simulink model "Rebuild"  (R2024b)
settings: Solver=VariableStepAuto  StartTime=0.0  StopTime=12  RelTol=1e-3
values from neighbouring files (symbols this model uses):
  A = 1.1    [RT14e_Parameters.m]    (also in RT15e_Parameters.m = 1.088; RT15evo_Parameters.m = 1.088)
  Aero_balance = 55    [RT14e_Parameters.m]    (also in RT15e_Parameters.m; RT15evo_Parameters.m)
  Aeromaps_ON = 0    [SIM_setup.m]
  air_density = 1.2    [SIM_setup.m]
  Balance_FW = Data_FW_STD(1:end,2)    [RT15e_Parameters.m]    (also in RT15evo_Parameters.m)
  Balance_R_11 = Data_R_11(1:end,2)    [RT15e_Parameters.m]    (also in RT15evo_Parameters.m)
  Br_coef_of_friction_F = 0.33    [RT14e_Parameters.m]    (also in RT15e_Parameters.m; RT15evo_Parameters.m)
  Br_coef_of_friction_R = 0.33    [RT14e_Parameters.m]    (also in RT15e_Parameters.m; RT15evo_Parameters.m)
  Br_pistons_area_F = 3617.26/1e6    (= 0.00361726)    [RT14e_Parameters.m]    (also in RT15e_Parameters.m; RT15evo_Parameters.m)
  Br_pistons_area_R = 2026.83/1e6    (= 0.00202683)    [RT14e_Parameters.m]    (also in RT15e_Parameters.m; RT15evo_Parameters.m)
  CdA = 1.31*A    (= 1.441)    [RT14e_Parameters.m]    (also in RT15e_Parameters.m = 1.700544; RT15evo_Parameters.m = 1.700544)
  CdA_FW = Data_FW_STD(1:end,3)    [RT15e_Parameters.m]    (also in RT15evo_Parameters.m)
  CdA_R_11 = Data_R_11(1:end,3)    [RT15e_Parameters.m]    (also in RT15evo_Parameters.m)
  ClA = 3.3*A    (= 3.63)    [RT14e_Parameters.m]    (also in RT15e_Parameters.m = 4.36288; RT15evo_Parameters.m = 4.36288)
  ClA_FW = Data_FW_STD(1:end,4)    [RT15e_Parameters.m]    (also in RT15evo_Parameters.m)
  ClA_R_11 = Data_R_11(1:end,4)    [RT15e_Parameters.m]    (also in RT15evo_Parameters.m)
  CoG_z = 0.35    [RT14e_Parameters.m]    (also in RT15e_Parameters.m = 0.28495; RT15evo_Parameters.m = 0.28495)
  Default_Fz_FL = Default_Fz_F/2 + (Default_Fz_F*CoG_y/Track_Front)    [RT14e_Parameters.m]    (also in RT15e_Parameters.m; RT15evo_Parameters.m)
  Default_Fz_FR = Default_Fz_F/2 - (Default_Fz_F*CoG_y/Track_Front)    [RT14e_Parameters.m]    (also in RT15e_Parameters.m; RT15evo_Parameters.m)
  Default_Fz_RL = Default_Fz_R/2 + (Default_Fz_R*CoG_y/Track_Rear)    [RT14e_Parameters.m]    (also in RT15e_Parameters.m; RT15evo_Parameters.m)
  Default_Fz_RR = Default_Fz_R/2 - (Default_Fz_R*CoG_y/Track_Rear)    [RT14e_Parameters.m]    (also in RT15e_Parameters.m; RT15evo_Parameters.m)
  Effective_br_disk_r_F = 0.0905    [RT14e_Parameters.m]    (also in RT15e_Parameters.m; RT15evo_Parameters.m)
  Effective_br_disk_r_R = 0.0895    [RT14e_Parameters.m]    (also in RT15e_Parameters.m; RT15evo_Parameters.m)
  Front_brake_balance = 0.0    (= 0)    [RT14e_Parameters.m]    (also in RT15e_Parameters.m; RT15evo_Parameters.m)
  Front_brake_pump_area = 153.94    [RT14e_Parameters.m]    (also in RT15e_Parameters.m; RT15evo_Parameters.m)
  Front_desired_brake_p_balance = 0.6    [RT14e_Parameters.m]    (also in RT15e_Parameters.m; RT15evo_Parameters.m)
  FW_Setup = Data_FW_STD(1:end,1)    [RT15e_Parameters.m]    (also in RT15evo_Parameters.m)
  Fx = Data_Fx(2:end,3:end)    [RT14e_Parameters.m]    (also in RT15e_Parameters.m; RT15evo_Parameters.m)
  Fy = Data_Fy(2:end,3:end)    [RT14e_Parameters.m]    (also in RT15e_Parameters.m; RT15evo_Parameters.m)
  Fz = Data_Fy(2:end,2)    [RT14e_Parameters.m]    (also in RT15e_Parameters.m; RT15evo_Parameters.m)
  g = 9.81    [SIM_setup.m]
  Gear_ratio = 12.9    [RT14e_Parameters.m]    (also in RT15e_Parameters.m; RT15evo_Parameters.m)
  Iz_wehicle = 120    [RT14e_Parameters.m]    (also in RT15e_Parameters.m; RT15evo_Parameters.m)
  Iz_wheel = 0.15    [RT14e_Parameters.m]    (also in RT15e_Parameters.m; RT15evo_Parameters.m)
  Lf = Wheelbase - CoG_x    (= 0.77)    [RT14e_Parameters.m]    (also in RT15e_Parameters.m = 0.7504; RT15evo_Parameters.m = 0.7504)
  LLTD = 0.45    [RT14e_Parameters.m]    (also in RT15e_Parameters.m = 0.55; RT15evo_Parameters.m = 0.55)
  Lock_brake_balance = false    [RT14e_Parameters.m]    (also in RT15e_Parameters.m; RT15evo_Parameters.m)
  Lr = Wheelbase - Lf    (= 0.755)    [RT14e_Parameters.m]    (also in RT15e_Parameters.m = 0.7746; RT15evo_Parameters.m = 0.7746)
  Mass = Vehicle_mass + Driver_mass    (= 290)    [RT14e_Parameters.m]    (also in RT15e_Parameters.m = 265; RT15evo_Parameters.m)
  Motor_maximum_power = 35366    [RT14e_Parameters.m]    (also in RT15e_Parameters.m; RT15evo_Parameters.m)
  RB_torque_setting_1 = -2    [RT14e_Parameters.m]    (also in RT15e_Parameters.m; RT15evo_Parameters.m)
  RB_torque_setting_10 = -20    [RT14e_Parameters.m]    (also in RT15e_Parameters.m; RT15evo_Parameters.m)
  RB_torque_setting_2 = -4    [RT14e_Parameters.m]    (also in RT15e_Parameters.m; RT15evo_Parameters.m)
  RB_torque_setting_3 = -6    [RT14e_Parameters.m]    (also in RT15e_Parameters.m; RT15evo_Parameters.m)
  RB_torque_setting_4 = -8    [RT14e_Parameters.m]    (also in RT15e_Parameters.m; RT15evo_Parameters.m)
  RB_torque_setting_5 = -10    [RT14e_Parameters.m]    (also in RT15e_Parameters.m; RT15evo_Parameters.m)
  RB_torque_setting_6 = -12    [RT14e_Parameters.m]    (also in RT15e_Parameters.m; RT15evo_Parameters.m)
  RB_torque_setting_7 = -14    [RT14e_Parameters.m]    (also in RT15e_Parameters.m; RT15evo_Parameters.m)
  RB_torque_setting_8 = -16    [RT14e_Parameters.m]    (also in RT15e_Parameters.m; RT15evo_Parameters.m)
  RB_torque_setting_9 = -18    [RT14e_Parameters.m]    (also in RT15e_Parameters.m; RT15evo_Parameters.m)
  Rear_brake_pump_area = 198.56    [RT14e_Parameters.m]    (also in RT15e_Parameters.m; RT15evo_Parameters.m)
  Roll_Angle_11 = Data_R_11(1:end,1)    [RT15e_Parameters.m]    (also in RT15evo_Parameters.m)
  SA = Data_Fy(1,3:end)    [RT14e_Parameters.m]    (also in RT15e_Parameters.m; RT15evo_Parameters.m)
  SR = Data_Fx(1,3:end)    [RT14e_Parameters.m]    (also in RT15e_Parameters.m; RT15evo_Parameters.m)
  start_acc_x = double(start_acc_x_ts.Data)    [SIM_setup.m]
  start_acc_y = double(start_acc_y_ts.Data)    [SIM_setup.m]
  start_time = 1188    [SIM_setup.m]
  start_velocity_x = double(start_velocity_x_ts.Data)    [SIM_setup.m]
  start_velocity_y = double(start_velocity_y_ts.Data)    [SIM_setup.m]
  start_yaw_acc = double(start_yaw_acc_ts.Data)    [SIM_setup.m]
  start_yaw_rate = double(start_yaw_rate_ts.Data)    [SIM_setup.m]
  Static_Camber_FL = 0    [RT14e_Parameters.m]    (also in RT15e_Parameters.m; RT15evo_Parameters.m)
  Static_Camber_FR = 0    [RT14e_Parameters.m]    (also in RT15e_Parameters.m; RT15evo_Parameters.m)
  Static_Camber_RL = 0    [RT14e_Parameters.m]    (also in RT15e_Parameters.m; RT15evo_Parameters.m)
  Static_Camber_RR = 0    [RT14e_Parameters.m]    (also in RT15e_Parameters.m; RT15evo_Parameters.m)
  Static_Toe_FL = 0    [RT14e_Parameters.m]    (also in RT15e_Parameters.m; RT15evo_Parameters.m)
  Static_Toe_FR = 0    [RT14e_Parameters.m]    (also in RT15e_Parameters.m; RT15evo_Parameters.m)
  Static_Toe_RL = 0    [RT14e_Parameters.m]    (also in RT15e_Parameters.m; RT15evo_Parameters.m)
  Static_Toe_RR = 0    [RT14e_Parameters.m]    (also in RT15e_Parameters.m; RT15evo_Parameters.m)
  Steering_Angle_FL = Data_Steering(1:end,2)    [RT14e_Parameters.m]    (also in RT15e_Parameters.m; RT15evo_Parameters.m)
  Steering_Angle_FR = Data_Steering(1:end,3)    [RT14e_Parameters.m]    (also in RT15e_Parameters.m; RT15evo_Parameters.m)
  Steering_Wheel_Angle = Data_Steering(1:end,1)    [RT14e_Parameters.m]    (also in RT15e_Parameters.m; RT15evo_Parameters.m)
  Tire_radius = 0.203    [RT14e_Parameters.m]    (also in RT15e_Parameters.m; RT15evo_Parameters.m)
  Torque_limit_2 = Motor_maximum_torque*0.2    (= 5.82)    [RT14e_Parameters.m]    (also in RT15e_Parameters.m; RT15evo_Parameters.m)
  Torque_limit_3 = Motor_maximum_torque*0.3    (= 8.73)    [RT14e_Parameters.m]    (also in RT15e_Parameters.m; RT15evo_Parameters.m)
  Torque_limit_4 = Motor_maximum_torque*0.4    (= 11.64)    [RT14e_Parameters.m]    (also in RT15e_Parameters.m; RT15evo_Parameters.m)
  Torque_limit_5 = Motor_maximum_torque*0.5    (= 14.55)    [RT14e_Parameters.m]    (also in RT15e_Parameters.m; RT15evo_Parameters.m)
  Torque_limit_6 = Motor_maximum_torque*0.6    (= 17.46)    [RT14e_Parameters.m]    (also in RT15e_Parameters.m; RT15evo_Parameters.m)
  Torque_limit_7 = Motor_maximum_torque*0.7    (= 20.37)    [RT14e_Parameters.m]    (also in RT15e_Parameters.m; RT15evo_Parameters.m)
  Torque_limit_8 = Motor_maximum_torque*0.8    (= 23.28)    [RT14e_Parameters.m]    (also in RT15e_Parameters.m; RT15evo_Parameters.m)
  Torque_limit_9 = 29.1    [RT14e_Parameters.m]    (also in RT15e_Parameters.m; RT15evo_Parameters.m)
  Torque_limit_max = Motor_maximum_torque    (= 29.1)    [RT14e_Parameters.m]    (also in RT15e_Parameters.m; RT15evo_Parameters.m)
  Torque_limit_min = Motor_maximum_torque*0.1    (= 2.91)    [RT14e_Parameters.m]    (also in RT15e_Parameters.m; RT15evo_Parameters.m)
  Torque_limit_set = 10    [RT14e_Parameters.m]    (also in RT15e_Parameters.m; RT15evo_Parameters.m)
  Track_Front = 1.2    [RT14e_Parameters.m]    (also in RT15e_Parameters.m; RT15evo_Parameters.m)
  Track_Rear = 1.18    [RT14e_Parameters.m]    (also in RT15e_Parameters.m; RT15evo_Parameters.m)
  TV_ON = 0    [SIM_setup.m]
  TV_RB_understeer_gradient_1 = -0.5    [RT14e_Parameters.m]    (also in RT15e_Parameters.m; RT15evo_Parameters.m)
  TV_RB_understeer_gradient_10 = 0.005    [RT14e_Parameters.m]    (also in RT15e_Parameters.m; RT15evo_Parameters.m)
  TV_RB_understeer_gradient_2 = -0.1    [RT14e_Parameters.m]    (also in RT15e_Parameters.m; RT15evo_Parameters.m)
  TV_RB_understeer_gradient_3 = 0.08    [RT14e_Parameters.m]    (also in RT15e_Parameters.m; RT15evo_Parameters.m)
  TV_RB_understeer_gradient_4 = 0.06    [RT14e_Parameters.m]    (also in RT15e_Parameters.m; RT15evo_Parameters.m)
  TV_RB_understeer_gradient_5 = 0.05    [RT14e_Parameters.m]    (also in RT15e_Parameters.m; RT15evo_Parameters.m)
  TV_RB_understeer_gradient_6 = 0.04    [RT14e_Parameters.m]    (also in RT15e_Parameters.m; RT15evo_Parameters.m)
  TV_RB_understeer_gradient_7 = 0.03    [RT14e_Parameters.m]    (also in RT15e_Parameters.m; RT15evo_Parameters.m)
  TV_RB_understeer_gradient_8 = 0.02    [RT14e_Parameters.m]    (also in RT15e_Parameters.m; RT15evo_Parameters.m)
  TV_RB_understeer_gradient_9 = 0.01    [RT14e_Parameters.m]    (also in RT15e_Parameters.m; RT15evo_Parameters.m)
  TV_understeer_gradient_1 = -0.5    [RT14e_Parameters.m]    (also in RT15e_Parameters.m; RT15evo_Parameters.m)
  TV_understeer_gradient_10 = 0.002    [RT14e_Parameters.m]    (also in RT15e_Parameters.m; RT15evo_Parameters.m)
  TV_understeer_gradient_2 = -0.1    [RT14e_Parameters.m]    (also in RT15e_Parameters.m; RT15evo_Parameters.m)
  TV_understeer_gradient_3 = 0.06    [RT14e_Parameters.m]    (also in RT15e_Parameters.m; RT15evo_Parameters.m)
  TV_understeer_gradient_4 = 0.05    [RT14e_Parameters.m]    (also in RT15e_Parameters.m; RT15evo_Parameters.m)
  TV_understeer_gradient_5 = 0.04    [RT14e_Parameters.m]    (also in RT15e_Parameters.m; RT15evo_Parameters.m)
  TV_understeer_gradient_6 = 0.03    [RT14e_Parameters.m]    (also in RT15e_Parameters.m; RT15evo_Parameters.m)
  TV_understeer_gradient_7 = 0.02    [RT14e_Parameters.m]    (also in RT15e_Parameters.m; RT15evo_Parameters.m)
  TV_understeer_gradient_8 = 0.01    [RT14e_Parameters.m]    (also in RT15e_Parameters.m; RT15evo_Parameters.m)
  TV_understeer_gradient_9 = 0.005    [RT14e_Parameters.m]    (also in RT15e_Parameters.m; RT15evo_Parameters.m)
  Vx_APPS_ON = 1    [SIM_setup.m]
  Wheel_rolling_resistance = 0.055    [RT14e_Parameters.m]    (also in RT15e_Parameters.m; RT15evo_Parameters.m)
  Wheelbase = 1.525    [RT14e_Parameters.m]    (also in RT15e_Parameters.m; RT15evo_Parameters.m)
undefined symbols (not defined in the file or in its folder): Actual_Torque_Value_RL, Actual_Torque_Value_RR, aero_balance, APPS, Brake_Pressure_Front, Brake_Pressure_Rear, Cl, lateral_load_transfer_distribution, maths_GPS_Velocity, Max_Torque, rad, s, Steering_position, tire_radius, wheel_base, Wheel_Speed_RL, Wheel_Speed_RR, Xsens_MTI_670_accX, Xsens_MTI_670_accY, Xsens_MTI_670_gyrZ
libraries: simulink x30, simulink_extras x11, slpidlib x9, dspstat3 x4, slrealtimeloglib x1, aerolibconvert2 x1
(part 1 of 6)
settings Model: Creator=ciech  LastModifiedBy=ciech
settings SolverCC: ZeroCrossControl=EnableAll
settings DebuggingCC: IgnoredZcDiagnostic=none

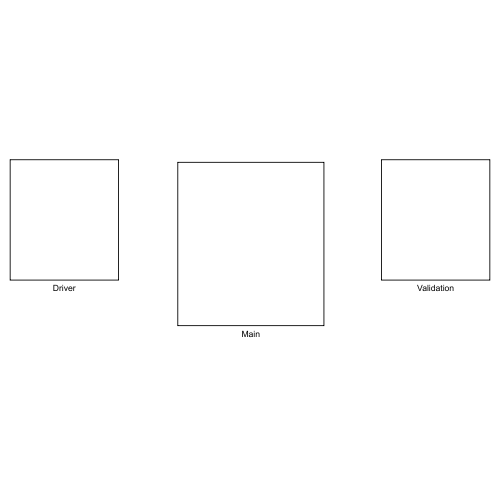
[thumbnail: Simulink's stored preview of the top-level diagram]
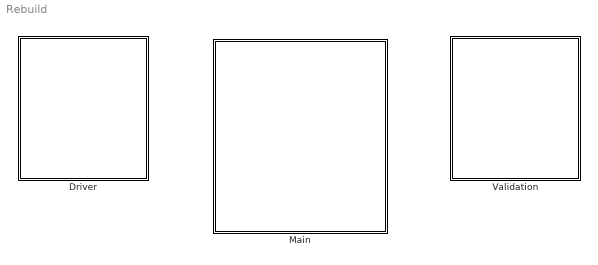
== system Rebuild ==
  Driver : Subsystem
  Main : Subsystem
  Validation : Subsystem

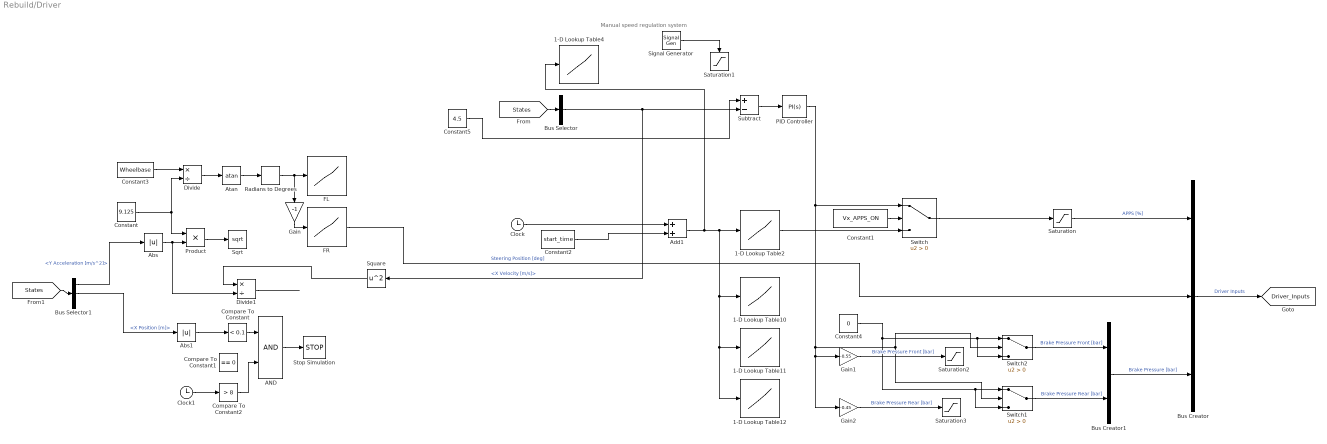
== system Rebuild/Driver ==
  note: Manual speed regulation system
  1-D Lookup Table10 : Lookup_n-D  NumberOfTableDimensions=1  BreakpointsForDimension1=Steering_position.Time  Table=Steering_position.Value  InternalRulePriority=Speed  RndMeth=Simplest
  1-D Lookup Table11 : Lookup_n-D  NumberOfTableDimensions=1  BreakpointsForDimension1=Brake_Pressure_Front.Time  Table=Brake_Pressure_Front.Value  InternalRulePriority=Speed  RndMeth=Simplest
  1-D Lookup Table12 : Lookup_n-D  NumberOfTableDimensions=1  BreakpointsForDimension1=Brake_Pressure_Rear.Time  Table=Brake_Pressure_Rear.Value  InternalRulePriority=Speed  RndMeth=Simplest
  1-D Lookup Table2 : Lookup_n-D  NumberOfTableDimensions=1  BreakpointsForDimension1=APPS.Time  Table=APPS.Value  InternalRulePriority=Speed  RndMeth=Simplest
  1-D Lookup Table4 : Lookup_n-D  NumberOfTableDimensions=1  BreakpointsForDimension1=maths_GPS_Velocity.Time  Table=maths_GPS_Velocity.Value  InternalRulePriority=Speed  RndMeth=Simplest
  AND : Logic  IconShape=distinctive  AllPortsSameDT=off  OutDataTypeStr=boolean
  Abs : Abs  SaturateOnIntegerOverflow=off
  Abs1 : Abs  SaturateOnIntegerOverflow=off
  Add1 : Sum
  Atan : Trigonometry  Operator=atan
  Bus Creator : BusCreator  Inputs=3
  Bus Creator1 : BusCreator  Inputs=2
  Bus Selector : BusSelector  OutputSignals=Velocitiy [m/s].X Velocity [m/s]
  Bus Selector1 : BusSelector  OutputSignals=Acceleration [m/s].Y Acceleration [m/s^2],Position [m].X Position [m],Position [m].Y Position [m]
  Clock : Clock
  Clock1 : Clock
  Compare To Constant : simulink/Logic and Bit Operations/Compare To Constant  relop=<  const=0.1  OutDataTypeStr=boolean
  Compare To Constant1 : simulink/Logic and Bit Operations/Compare To Constant  relop===  const=0  OutDataTypeStr=boolean
  Compare To Constant2 : simulink/Logic and Bit Operations/Compare To Constant  relop=>  const=8  OutDataTypeStr=boolean
  Constant : Constant  Value=9.125
  Constant1 : Constant  Value=Vx_APPS_ON
  Constant2 : Constant  Value=start_time
  Constant3 : Constant  Value=Wheelbase
  Constant4 : Constant  Value=0
  Constant5 : Constant  Value=4.5
  Divide : Product  Inputs=*/
  Divide1 : Product  Inputs=*/
  FL : Lookup_n-D  NumberOfTableDimensions=1  BreakpointsForDimension1=Steering_Angle_FL  Table=Steering_Wheel_Angle  InternalRulePriority=Speed  RndMeth=Simplest
  FR : Lookup_n-D  NumberOfTableDimensions=1  BreakpointsForDimension1=Steering_Angle_FR*-1  Table=Steering_Wheel_Angle  InternalRulePriority=Speed  RndMeth=Simplest
  Gain : Gain  Gain=-1
  Gain1 : Gain  Gain=-0.55
  Gain2 : Gain  Gain=-0.45
  PID Controller : slpidlib/PID Controller  Controller=PI  Form=Parallel  TimeDomain=Continuous-time  UseExternalTs=off  SampleTime=-1  IntegratorMethod=Forward Euler  FilterMethod=Forward Euler  ControllerParametersSource=internal  P=70  I=40  UseKiTs=off  D=20  UseExternalDerivativeSource=off  N=100  UseFilter=on  TunerSelectOption=Transfer Function Based (PID Tuner App)  InitialConditionSource=internal  InitialConditionForIntegrator=0  InitialConditionForFilter=0  DifferentiatorICPrevScaledInput=0  ExternalReset=none  TrackingMode=off  Kt=1  LimitOutput=off  SatLimitsSource=internal  UpperSaturationLimit=100  LowerSaturationLimit=0  LinearizeAsGain=on  AntiWindupMode=back-calculation  Kb=1  LimitIntegrator=off  UpperIntegratorSaturationLimit=inf  LowerIntegratorSaturationLimit=-inf  POutMin=[]  POutMax=[]  IOutMin=[]  IOutMax=[]  DOutMin=[]  DOutMax=[]  NOutMin=[]  NOutMax=[]  SumOutMin=[]  SumOutMax=[]  SaturationOutMin=[]  SaturationOutMax=[]  PParamMin=[]  PParamMax=[]  IParamMin=[]  IParamMax=[]  DParamMin=[]  DParamMax=[]  NParamMin=[]  NParamMax=[]  KbParamMin=[]  KbParamMax=[]  KtParamMin=[]  KtParamMax=[]  KbOutMin=[]  KbOutMax=[]  KtOutMin=[]  KtOutMax=[]  IntegratorOutMin=[]  IntegratorOutMax=[]  FilterOutMin=[]  FilterOutMax=[]  SumI1OutMin=[]  SumI1OutMax=[]  SumI2OutMin=[]  SumI2OutMax=[]  SumI3OutMin=[]  SumI3OutMax=[]  SumI4OutMin=[]  SumI4OutMax=[]  SumDOutMin=[]  SumDOutMax=[]  DifferentiatorOutMin=[]  DifferentiatorOutMax=[]  FilterDiffOutCoefMin=[]  FilterDiffOutCoefMax=[]  ReciprocalOutMin=[]  ReciprocalOutMax=[]  SumDenOutMin=[]  SumDenOutMax=[]  SumNumOutMin=[]  SumNumOutMax=[]  DivideOutMin=[]  DivideOutMax=[]  UdiffTsProdOutMin=[]  UdiffTsProdOutMax=[]  NTsProdOutMin=[]  NTsProdOutMax=[]  UintegralTsProdOutMin=[]  UintegralTsProdOutMax=[]  UngainTsProdOutMin=[]  UngainTsProdOutMax=[]  ClampingZeroOutDataTypeStr=Inherit: Inherit via back propagation  ClampingZeroOutMin=[]  ClampingZeroOutMax=[]  FilterDenConstantOutDataTypeStr=Inherit: Inherit via back propagation  FilterDenConstantOutMin=[]  FilterDenConstantOutMax=[]  PCopyOutDataTypeStr=Inherit: Inherit via back propagation  PCopyOutMin=[]  PCopyOutMax=[]  NCopyOutDataTypeStr=Inherit: Inherit via back propagation  NCopyOutMin=[]  NCopyOutMax=[]  IntegratorContinuousStateAttributes=''  IntegratorStateMustResolveToSignalObject=off  IntegratorRTWStateStorageClass=Auto  FilterContinuousStateAttributes=''  FilterStateMustResolveToSignalObject=off  FilterRTWStateStorageClass=Auto  ParallelPVariant=InternalParameters  IdealPVariant=Disabled  IVariant=InternalParameters  DVariant=Disabled  IntegratorVariant=Continuous  SatVariant=Disabled  AWVariant=Passthrough  PCopyVariant=Disabled  TRVariant=Disabled  FdbkBlocksVariant=Forward  IdealPFdbkVariant=Disabled  SatFdbkVariant=Disabled  DerivativeFilterVariant=Disabled  NVariant=Disabled  NCopyVariant=Disabled_SignalSpec  FilterICVariant=Disabled  IntegratorICVariant=InternalICs  ExternalResetVariant=Disabled  TRSumVariant=Passthrough  SumFdbkVariant=Disabled  SumVariant=Sum_PI  TsampFilterVariant=InternalTs  TsampNgainVariant=Passthrough  TsampIntegralVariant=Disabled_SignalSpec  ExternalSaturationOutDataTypeStr=Inherit: Same as second input  DerivativeSourceVariant=Disabled  PreIntVariant=InternalPreInt
  Product : Product
  Radians to Degrees : simulink_extras/Transformations/Radians to Degrees
  Saturation : Saturate  UpperLimit=100  LowerLimit=0
  Saturation1 : Saturate  UpperLimit=inf  LowerLimit=10
  Saturation2 : Saturate  UpperLimit=70  LowerLimit=0
  Saturation3 : Saturate  UpperLimit=70  LowerLimit=0
  Signal Generator : SignalGenerator  Amplitude=20  Frequency=2  Units=rad/sec
  Sqrt : Sqrt
  Square : Math  Operator=square
  Stop Simulation : Stop
  Subtract : Sum  Inputs=+-
  Switch : Switch  Criteria=u2 > Threshold  SaturateOnIntegerOverflow=off  InputSameDT=off
  Switch1 : Switch  Criteria=u2 > Threshold  SaturateOnIntegerOverflow=off  InputSameDT=off
  Switch2 : Switch  Criteria=u2 > Threshold  SaturateOnIntegerOverflow=off  InputSameDT=off
  tag scope: Driver_Inputs=global
  wires:
  Saturation/1 -> Bus Creator/1  "APPS [%]"
  Clock/1 -> Add1/1
  Bus Creator1/1 -> Bus Creator/3  "Brake Pressure [bar]"
  Switch2/1 -> Bus Creator1/1  "Brake Pressure Front [bar]"
  Switch1/1 -> Bus Creator1/2  "Brake Pressure Rear [bar]"
  Constant2/1 -> Add1/2
  Add1/1 -> 1-D Lookup Table4/1, 1-D Lookup Table12/1, 1-D Lookup Table11/1, 1-D Lookup Table10/1, 1-D Lookup Table2/1
  Bus Selector/1 -> Square/1, Subtract/2  "<X Velocity [m/s]>"
  Subtract/1 -> PID Controller/1
  [States] -> Bus Selector/1
  1-D Lookup Table2/1 -> Switch/3
  Constant1/1 -> Switch/2
  Bus Creator/1 -> [Driver_Inputs]  "Driver Inputs"
  Switch/1 -> Saturation/1
  PID Controller/1 -> Switch1/2, Switch2/2, Gain1/1, Gain2/1, Switch/1
  Constant3/1 -> Divide/1
  Constant/1 -> Product/1, Divide/2
  Divide/1 -> Atan/1
  Atan/1 -> Radians to Degrees/1
  [States] -> Bus Selector1/1
  Bus Selector1/1 -> Abs/1  "<Y Acceleration [m/s^2]>"
  Product/1 -> Sqrt/1
  Signal Generator/1 -> Saturation1/1
  Abs/1 -> Divide1/2, Product/2
  Radians to Degrees/1 -> FL/1, Gain/1
  Square/1 -> Divide1/1
  Gain/1 -> FR/1
  Compare To Constant/1 -> AND/1
  Compare To Constant2/1 -> AND/2
  Clock1/1 -> Compare To Constant2/1
  Abs1/1 -> Compare To Constant/1
  Bus Selector1/2 -> Abs1/1  "<X Position [m]>"
  Constant4/1 -> Switch1/3, Switch1/1, Switch2/3, Switch2/1
  Gain1/1 -> Saturation2/1  "Brake Pressure Front [bar]"
  Gain2/1 -> Saturation3/1  "Brake Pressure Rear [bar]"
  Divide1/1 -> ?
  FR/1 -> Bus Creator/2  "Steering Position [deg]"
  AND/1 -> Stop Simulation/1
  Constant5/1 -> Subtract/1

== system Rebuild/Main ==
  Aero : Subsystem
      mask Display: image('aero_rt15.png');
  Chassis : Subsystem
      mask Display: image('monocoque.png');
  Powertrain : Subsystem
      mask Display: image('PRT.png');
  Suspension : Subsystem
      mask Display: image('sus.png');
  Wheels & Tires : Subsystem
      mask Display: image('wheel_rt15e.png');

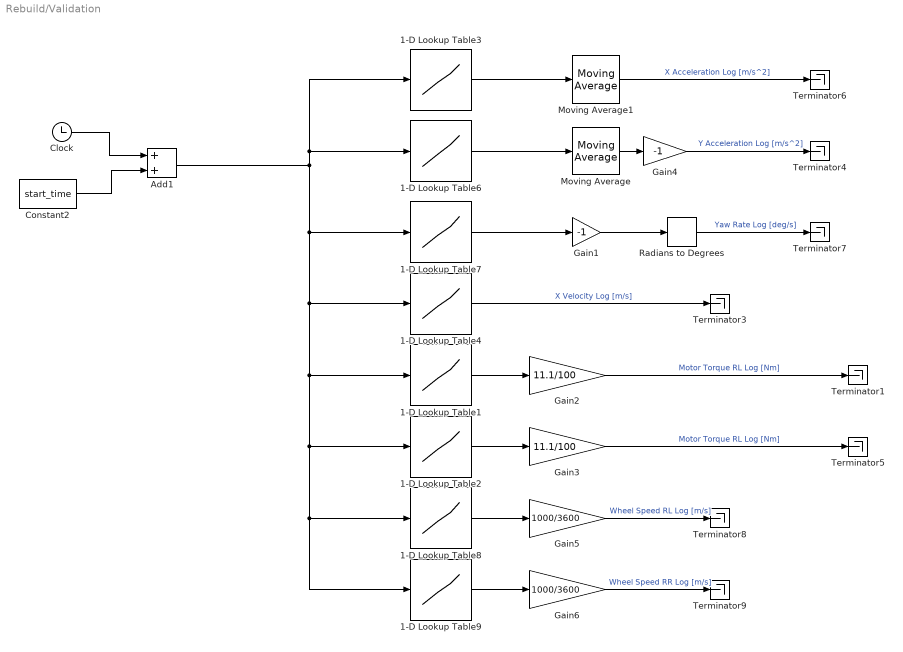
== system Rebuild/Validation ==
  1-D Lookup Table1 : Lookup_n-D  NumberOfTableDimensions=1  BreakpointsForDimension1=Actual_Torque_Value_RL.Time  Table=Actual_Torque_Value_RL.Value  InternalRulePriority=Speed  RndMeth=Simplest
  1-D Lookup Table2 : Lookup_n-D  NumberOfTableDimensions=1  BreakpointsForDimension1=Actual_Torque_Value_RR.Time  Table=Actual_Torque_Value_RR.Value  InternalRulePriority=Speed  RndMeth=Simplest
  1-D Lookup Table3 : Lookup_n-D  NumberOfTableDimensions=1  BreakpointsForDimension1=Xsens_MTI_670_accX.Time  Table=Xsens_MTI_670_accX.Value  InternalRulePriority=Speed  RndMeth=Simplest
  1-D Lookup Table4 : Lookup_n-D  NumberOfTableDimensions=1  BreakpointsForDimension1=maths_GPS_Velocity.Time  Table=maths_GPS_Velocity.Value  InternalRulePriority=Speed  RndMeth=Simplest
  1-D Lookup Table6 : Lookup_n-D  NumberOfTableDimensions=1  BreakpointsForDimension1=Xsens_MTI_670_accY.Time  Table=Xsens_MTI_670_accY.Value  InternalRulePriority=Speed  RndMeth=Simplest
  1-D Lookup Table7 : Lookup_n-D  NumberOfTableDimensions=1  BreakpointsForDimension1=Xsens_MTI_670_gyrZ.Time  Table=Xsens_MTI_670_gyrZ.Value  InternalRulePriority=Speed  RndMeth=Simplest
  1-D Lookup Table8 : Lookup_n-D  NumberOfTableDimensions=1  BreakpointsForDimension1=Wheel_Speed_RL.Time  Table=Wheel_Speed_RL.Value  InternalRulePriority=Speed  RndMeth=Simplest
  1-D Lookup Table9 : Lookup_n-D  NumberOfTableDimensions=1  BreakpointsForDimension1=Wheel_Speed_RR.Time  Table=Wheel_Speed_RR.Value  InternalRulePriority=Speed  RndMeth=Simplest
  Add1 : Sum
  Clock : Clock
  Constant2 : Constant  Value=start_time
  Gain1 : Gain  Gain=-1
  Gain2 : Gain  Gain=11.1/100
  Gain3 : Gain  Gain=11.1/100
  Gain4 : Gain  Gain=-1
  Gain5 : Gain  Gain=1000/3600
  Gain6 : Gain  Gain=1000/3600
  Moving Average : dspstat3/Moving Average  Method=Sliding window  ForgettingFactorPort=off  SpecifyWindowLength=on  WindowLength=50  OverlapLength=49  AllowArbitraryInputLength=off  ForgettingFactor=0.9  SimulateUsing=Code generation
  Moving Average1 : dspstat3/Moving Average  Method=Sliding window  ForgettingFactorPort=off  SpecifyWindowLength=on  WindowLength=50  OverlapLength=49  AllowArbitraryInputLength=off  ForgettingFactor=0.9  SimulateUsing=Code generation
  Radians to Degrees : simulink_extras/Transformations/Radians to Degrees
  Terminator{1,3..9} (8 alike) : Terminator
  wires:
  1-D Lookup Table6/1 -> Moving Average/1
  Gain4/1 -> Terminator4/1  "Y Acceleration Log [m/s^2]"
  Moving Average/1 -> Gain4/1
  Add1/1 -> 1-D Lookup Table7/1, 1-D Lookup Table2/1, 1-D Lookup Table8/1, 1-D Lookup Table9/1, 1-D Lookup Table1/1, 1-D Lookup Table4/1, 1-D Lookup Table3/1, 1-D Lookup Table6/1
  Clock/1 -> Add1/1
  Constant2/1 -> Add1/2
  Gain3/1 -> Terminator5/1  "Motor Torque RL Log [Nm]"
  1-D Lookup Table3/1 -> Moving Average1/1
  Moving Average1/1 -> Terminator6/1  "X Acceleration Log [m/s^2]"
  1-D Lookup Table4/1 -> Terminator3/1  "X Velocity Log [m/s]"
  Radians to Degrees/1 -> Terminator7/1  "Yaw Rate Log [deg/s]"
  1-D Lookup Table7/1 -> Gain1/1
  Gain1/1 -> Radians to Degrees/1
  1-D Lookup Table1/1 -> Gain2/1
  1-D Lookup Table2/1 -> Gain3/1
  Gain5/1 -> Terminator8/1  "Wheel Speed RL Log [m/s]"
  1-D Lookup Table8/1 -> Gain5/1
  Gain6/1 -> Terminator9/1  "Wheel Speed RR Log [m/s]"
  1-D Lookup Table9/1 -> Gain6/1
  Gain2/1 -> Terminator1/1  "Motor Torque RL Log [Nm]"

== system Rebuild/Main/Aero ==
  Bus Creator : BusCreator  Inputs=3
  Constants Calculation : Subsystem
  Subsystem : Subsystem
  Total Aero Forces Calculation : Subsystem
  tag scope: Aero=global
  wires:
  Constants Calculation/1(Aero Constants) -> Bus Creator/3, Total Aero Forces Calculation/1(Aero Constants)  "Aero Constants"
  Total Aero Forces Calculation/1(Total Aero Forces [N]) -> Subsystem/1(Total Aero Forces [N]), Bus Creator/2  "Total Aero Forces [N]"
  Subsystem/1(Aero Wheel Loads [N]) -> Bus Creator/1  "Aero Wheel Loads [N]"
  Bus Creator/1 -> [Aero]  "Aerodynamics"

== system Rebuild/Main/Chassis ==
  Acceleration Calculation : Subsystem
  Bus Creator{,1..2,4} (4 alike) : BusCreator  Inputs=3
  Bus Selector : BusSelector  OutputSignals=Total Aero Forces [N].Drag [N]
  Bus Selector1 : BusSelector  OutputSignals=Tire Forces [N[.Fx [N],Tire Forces [N[.Fy [N]
  Bus Selector2 : BusSelector  OutputSignals=Steering Angle [rad]
  Position Calculation : Subsystem
  Velocitiy Calculation : Subsystem
  tag scope: States=global
  wires:
  Bus Creator/1 -> [States]
  Bus Creator2/1 -> Bus Creator/1  "Velocitiy [m/s]"
  Bus Creator1/1 -> Bus Creator/2  "Acceleration [m/s]"
  Acceleration Calculation/3(Yaw Acceleration) -> Velocitiy Calculation/3(Yaw Acceleration [rad/s^2]), Bus Creator1/3
  Velocitiy Calculation/1(X Velocity) -> Bus Creator2/1
  Velocitiy Calculation/2(Y Velocity) -> Bus Creator2/2
  Velocitiy Calculation/3(Yaw Rate) -> Bus Creator2/3
  Bus Selector/1 -> Acceleration Calculation/1(Drag [N])  "<Drag [N]>"
  Bus Selector1/1 -> Acceleration Calculation/3(Fx [N])  "<Fx [N]>"
  Bus Selector1/2 -> Acceleration Calculation/4(Fy [N])  "<Fy [N]>"
  Acceleration Calculation/1(X Acceleration) -> Bus Creator1/1, Velocitiy Calculation/1(X Acceleration [m/s^2])
  Acceleration Calculation/2(Y Acceleration) -> Velocitiy Calculation/2(Y Acceleration [m/s^2]), Bus Creator1/2
  Position Calculation/1(X Position) -> Bus Creator4/1
  Position Calculation/2(Y Position) -> Bus Creator4/2
  Bus Creator4/1 -> Bus Creator/3  "Position [m]"
  Position Calculation/3(Yaw angle) -> Bus Creator4/3
  [Aero] -> Bus Selector/1
  [Tires] -> Bus Selector1/1
  [Sus] -> Bus Selector2/1
  Bus Selector2/1 -> Acceleration Calculation/2(Steering Angle [rad])  "<Steering Angle [rad]>"

== system Rebuild/Main/Powertrain ==
  Bus Creator : BusCreator  Inputs=1
  Energy Calculation : Subsystem
  Motors : Subsystem
  tag scope: PRT=global
  wires:
  Motors/1(Motor Torque [Nm]) -> Bus Creator/1  "Motor Torque [Nm]"
  Bus Creator/1 -> [PRT]
  Motors/2(Motor Power [W]) -> Energy Calculation/1(Motor Power [W])  "Motor Power [W]"

== system Rebuild/Main/Suspension ==
  Bus Creator : BusCreator  Inputs=3
  Kinematics : Subsystem
  Load Transfer : Subsystem
  Steering : Subsystem
  tag scope: Sus=global
  wires:
  Steering/1(Steering) -> Bus Creator/1
  Load Transfer/1(Load Transfer [N]) -> Bus Creator/2
  Kinematics/1(Kinematics) -> Bus Creator/3
  Bus Creator/1 -> [Sus]  "Suspension"

== system Rebuild/Main/Wheels & Tires ==
  Brakes : Subsystem
  Bus Creator : BusCreator  Inputs=3
  Bus Creator1 : BusCreator  Inputs=3
  Bus Creator3 : BusCreator  Inputs=2
  Bus Selector : BusSelector  OutputSignals=Tire Forces [N[.Fx [N],Tire Forces [N[.Fz [N]
  Bus Selector1 : BusSelector  OutputSignals=Motor Torque [Nm]
  Fx : Subsystem
  Fy : Subsystem
  Fz : Subsystem
  Slip Ratio & Slip Angle Calculation : Subsystem
  Wheel Speeds : Subsystem
      settings: PortSchema="{\"entries\":[{\"content\":{\"sides\":[{\"content\":{\"connectorIds\":[\"In1\",\"In2\",\"In3\"]},\"type\":\"ConnectorPlacement.EquallySpacedRectSide\",\"uuid\":\"124e436b-f64c-4028-8095-1d8f772c4fa3\"},{\"content\":{\"connectorIds\":[\"Out1\"],\"side\":\"RIGHT\"},\"type\":\"ConnectorPlacement.EquallySpacedRectSide\",\"uuid\":\"9f40d3b5-88bb-42e4-84dd-7d55a8f5d4b6\"},{\"content\":{\"connectorIds\":[\"In4\"],\"side\":\"TOP\"},\"type\":\"ConnectorPlacement.EquallySpacedRectSide\",\"uuid\":\"9d151df8-d681-4246-ac1a-4865a41edfc5\"}]},\"type\":\"ConnectorPlacement.EquallySpacedConnector\",\"uuid\":\"843c1e6a-deb6-4dbc-8d76-71cc70acac89\"}],\"packageUris\":[\"http://schema.mathworks.com/mf0/Connector/R2020b\"],\"version\":\"1.0\"}"
  tag scope: Tires=global
  wires:
  Slip Ratio & Slip Angle Calculation/1(Slip Ratio) -> Bus Creator3/1  "Slip Ratio"
  Slip Ratio & Slip Angle Calculation/2(Slip Angles [deg]) -> Bus Creator3/2  "Slip Angle [deg]"
  Fx/1(Fx [N]) -> Bus Creator/1  "Fx [N]"
  Fy/1(Fy [N]) -> Bus Creator/2  "Fy [N]"
  Bus Creator3/1 -> Fy/1(Slips), [Slips], Fx/1(Slips)  "Slips"
  Fz/1(Fz [N]) -> Bus Creator/3  "Fz [N]"
  Wheel Speeds/1(Wheel Speeds) -> [Wheel_Speeds], Slip Ratio & Slip Angle Calculation/1(Wheel Speeds [rad/s])  "Wheel Speeds"
  Bus Creator/1 -> Bus Creator1/1  "Tire Forces [N["
  [Tires] -> Bus Selector/1
  Bus Selector/2 -> Wheel Speeds/3(Fz [N])  "<Fz [N]>"
  Bus Selector/1 -> Wheel Speeds/2(Fx [N])  "<Fx [N]>"
  Brakes/1(Brake Torque [Nm]) -> Wheel Speeds/4(Brake Torque [Nm])  "Brake Torque [Nm]"
  [PRT] -> Bus Selector1/1
  Bus Selector1/1 -> Wheel Speeds/1(Motor Torque [Nm])  "<Motor Torque [Nm]>"
  Bus Creator1/1 -> [Tires]  "Tires"
  [Slips] -> Bus Creator1/2
  [Wheel_Speeds] -> Bus Creator1/3

== system Rebuild/Main/Aero/Constants Calculation ==
  Aero Balance : Lookup_n-D  Commented=on  NumberOfTableDimensions=1  BreakpointsForDimension1=Balance_R_11  Table=Roll_Angle_11  InternalRulePriority=Speed  RndMeth=Simplest
  Aero Balance1 : Lookup_n-D  Commented=on  NumberOfTableDimensions=1  BreakpointsForDimension1=Balance_FW  Table=FW_Setup  InternalRulePriority=Speed  RndMeth=Simplest
  Bus Creator : BusCreator  Inputs=3
  Bus Creator1 : BusCreator  Inputs=3
  Constant : Constant  Value=Aeromaps_ON
  Constant1 : Constant  Value=Aero_balance
  Constant2 : Constant  Value=CdA
  Constant3 : Constant  Value=ClA
  Downforce : Lookup_n-D  Commented=on  NumberOfTableDimensions=1  BreakpointsForDimension1=ClA_R_11  Table=Roll_Angle_11  InternalRulePriority=Speed  RndMeth=Simplest
  Downforce1 : Lookup_n-D  Commented=on  NumberOfTableDimensions=1  BreakpointsForDimension1=ClA_FW  Table=FW_Setup  InternalRulePriority=Speed  RndMeth=Simplest
  Drag : Lookup_n-D  Commented=on  NumberOfTableDimensions=1  BreakpointsForDimension1=CdA_R_11  Table=Roll_Angle_11  InternalRulePriority=Speed  RndMeth=Simplest
  Drag1 : Lookup_n-D  Commented=on  NumberOfTableDimensions=1  BreakpointsForDimension1=CdA_FW  Table=FW_Setup  InternalRulePriority=Speed  RndMeth=Simplest
  Switch : Switch  Criteria=u2 > Threshold  SaturateOnIntegerOverflow=off  InputSameDT=off
  Aero Constants : Outport
  wires:
  Drag/1 -> Bus Creator/1  "CdA"
  Aero Balance/1 -> Bus Creator/3  "Aero Balance [%]"
  Bus Creator1/1 -> Switch/3
  Constant/1 -> Switch/2
  Constant2/1 -> Bus Creator1/1  "CdA"
  Downforce/1 -> Bus Creator/2  "ClA"
  Constant3/1 -> Bus Creator1/2  "ClA"
  Constant1/1 -> Bus Creator1/3  "Aero Balance [%]"
  ? -> Downforce/1
  Bus Creator/1 -> Switch/1
  Switch/1 -> Aero Constants/1  "Aero Constants"
  ? -> Drag/1
  ? -> Aero Balance/1
  ? -> Aero Balance1/1
  ? -> Drag1/1
  ? -> Downforce1/1
  Drag1/1 -> ?  "CdA"

== system Rebuild/Main/Aero/Subsystem ==
  Total Aero Forces [N] : Inport
  Bus Creator : BusCreator  Inputs=4
  Bus Selector : BusSelector  OutputSignals=Downforce Front [N],Downforce Rear [N]
  Gain{1..4} (4 alike) : Gain  Gain=1/2
  Aero Wheel Loads [N] : Outport
  wires:
  Bus Selector/2 -> Gain4/1, Gain2/1  "<Downforce Rear [N]>"
  Bus Selector/1 -> Gain1/1, Gain3/1  "<Downforce Front [N]>"
  Bus Creator/1 -> Aero Wheel Loads [N]/1  "Aero Wheel Loads [N]"
  Total Aero Forces [N]/1 -> Bus Selector/1
  Gain3/1 -> Bus Creator/2  "Aero Load FR [N]"
  Gain4/1 -> Bus Creator/4  "Aero Load RR [N]"
  Gain2/1 -> Bus Creator/3  "Aero Load RL [N]"
  Gain1/1 -> Bus Creator/1  "Aero Load FL [N]"

== system Rebuild/Main/Aero/Total Aero Forces Calculation ==
  Aero Constants : Inport
  Bus Creator2 : BusCreator  Inputs=4
  Bus Selector : BusSelector  OutputSignals=Velocitiy [m/s].X Velocity [m/s]
  Bus Selector1 : BusSelector  OutputSignals=CdA,ClA,Aero Balance [%]
  Gain : Gain  Gain=0.01
  Gain1 : Gain  Gain=air_density
  Gain2 : Gain  Gain=1/2
  Product : Product
  Product1 : Product
  Product2 : Product
  Square : Math  Operator=square
  Subtract1 : Sum  Inputs=+-
  Total Aero Forces [N] : Outport
  wires:
  Aero Constants/1 -> Bus Selector1/1
  Bus Creator2/1 -> Total Aero Forces [N]/1  "Total Aero Forces [N]"
  Product/1 -> Bus Creator2/1  "Drag [N]"
  [States] -> Bus Selector/1
  Product2/1 -> Subtract1/2, Bus Creator2/4  "Downforce Front [N]"
  Gain1/1 -> Gain2/1
  Bus Selector1/2 -> Product1/2  "<ClA>"
  Bus Selector/1 -> Square/1  "<X Velocity [m/s]>"
  Bus Selector1/1 -> Product/1  "<CdA>"
  Subtract1/1 -> Bus Creator2/3  "Downforce Rear [N]"
  Square/1 -> Gain1/1
  Bus Selector1/3 -> Gain/1  "<Aero Balance [%]>"
  Product1/1 -> Product2/1, Bus Creator2/2, Subtract1/1  "Downforce [N]"
  Gain2/1 -> Product1/1, Product/2
  Gain/1 -> Product2/2

== system Rebuild/Main/Chassis/Acceleration Calculation ==
  Drag [N] : Inport
  Steering Angle [rad] : Inport  Port=2
  Fx [N] : Inport  Port=3
  Fy [N] : Inport  Port=4
  IC : InitialCondition  Value=start_yaw_acc
  IC1 : InitialCondition  Value=start_acc_y
  IC2 : InitialCondition  Value=start_acc_x
  Lateral_Acceleration : Subsystem
  Longitudinal Acceleration : Subsystem
  Memory : Memory  InheritSampleTime=on
  Memory1 : Memory  InheritSampleTime=on
  Memory2 : Memory  InheritSampleTime=on
  To Workspace1 : ToWorkspace  VariableName=Acc_Y  SaveFormat=Timeseries  SampleTime=-1
  To Workspace2 : ToWorkspace  VariableName=Acc_X  SaveFormat=Timeseries  SampleTime=-1
  To Workspace3 : ToWorkspace  VariableName=Acc_Yaw  SaveFormat=Timeseries  SampleTime=-1
  Yaw_Acceleration : Subsystem
  X Acceleration : Outport
  Y Acceleration : Outport  Port=2
  Yaw Acceleration : Outport  Port=3
  wires:
  Steering Angle [rad]/1 -> Lateral_Acceleration/1(Steering Angle [rad]), Yaw_Acceleration/1(Wheel_Angels [rad]), Longitudinal Acceleration/2(Steering Angle [rad])
  Fy [N]/1 -> Yaw_Acceleration/3(Y_Tire_Forces [N]), Lateral_Acceleration/3(Fy [N]), Longitudinal Acceleration/4(Fy [N])
  Fx [N]/1 -> Lateral_Acceleration/2(Fx [N]), Yaw_Acceleration/2(X_Tire_Forces [N]), Longitudinal Acceleration/3(Fx [N])
  Drag [N]/1 -> Longitudinal Acceleration/1(Drag [N])
  IC/1 -> To Workspace3/1, Yaw Acceleration/1  "Yaw Acceleration [rad/s^2]"
  IC1/1 -> To Workspace1/1, Y Acceleration/1  "Y Acceleration [m/s^2]"
  IC2/1 -> To Workspace2/1, X Acceleration/1  "X Acceleration [m/s^2]"
  Memory1/1 -> IC1/1
  Memory2/1 -> IC/1
  Memory/1 -> IC2/1
  Longitudinal Acceleration/1(X Acceleration [m/s^2]) -> Memory/1  "X Acceleration [m/s2]"
  Lateral_Acceleration/1(Y Acceleration [m/s^2]) -> Memory1/1  "Y Acceleration [m/s^2]"
  Yaw_Acceleration/1(Yaw_Acceleration [rad/s^2]) -> Memory2/1  "Yaw Acceleration [rad/s^2]"

== system Rebuild/Main/Chassis/Position Calculation ==
  Add : Sum
  Add1 : Sum
  Bus Selector : BusSelector  OutputSignals=Velocitiy [m/s].Yaw_Rate [rad/s],Velocitiy [m/s].X Velocity [m/s],Velocitiy [m/s].Y Velocity [m/s]
  Cos : Trigonometry  Operator=cos
  Gain : Gain  Gain=-1
  Integrator : Integrator
  Integrator5 : Integrator
  Integrator7 : Integrator
  Product{,1,4..5} (4 alike) : Product
  Sin : Trigonometry
  X Position : Outport
  Y Position : Outport  Port=2
  Yaw angle : Outport  Port=3
  wires:
  Integrator7/1 -> Y Position/1  "Y Position [m]"
  Integrator/1 -> Yaw angle/1, Sin/1, Cos/1  "Yaw angle [rad]"
  Integrator5/1 -> X Position/1  "X Position [m]"
  Product1/1 -> Add1/2
  Cos/1 -> Product5/2, Product1/1
  Sin/1 -> Product/2, Product4/2
  Add/1 -> Integrator5/1
  Bus Selector/3 -> Product1/2, Gain/1  "<Y Velocity [m/s]>"
  Product/1 -> Add1/1
  Gain/1 -> Product4/1
  Add1/1 -> Integrator7/1
  Product4/1 -> Add/2
  Product5/1 -> Add/1
  [States] -> Bus Selector/1
  Bus Selector/1 -> Integrator/1  "<Yaw_Rate [rad/s]>"
  Bus Selector/2 -> Product/1, Product5/1  "<X Velocity [m/s]>"

== system Rebuild/Main/Chassis/Velocitiy Calculation ==
  X Acceleration [m/s^2] : Inport
  Y Acceleration [m/s^2] : Inport  Port=2
  Yaw Acceleration [rad/s^2] : Inport  Port=3
  Add2 : Sum
  Integrator2 : Integrator  InitialCondition=start_velocity_y
  Integrator3 : Integrator  InitialCondition=start_velocity_x
  Integrator4 : Integrator  InitialCondition=start_yaw_rate
  Product2 : Product
  Product3 : Product
  Saturation : Saturate  UpperLimit=inf  LowerLimit=0.2
  Subtract1 : Sum  Inputs=-+
  To Workspace : ToWorkspace  VariableName=Vel_Y  SaveFormat=Timeseries  SampleTime=-1
  To Workspace1 : ToWorkspace  VariableName=Vel_X  SaveFormat=Timeseries  SampleTime=-1
  To Workspace2 : ToWorkspace  VariableName=Vel_Yaw  SaveFormat=Timeseries  SampleTime=-1
  X Velocity : Outport
  Y Velocity : Outport  Port=2
  Yaw Rate : Outport  Port=3
  wires:
  Yaw Acceleration [rad/s^2]/1 -> Integrator4/1
  Integrator2/1 -> To Workspace/1, [V_y], Y Velocity/1  "Y Velocity [m/s]"
  Product2/1 -> Add2/2
  Y Acceleration [m/s^2]/1 -> Subtract1/2
  Add2/1 -> Integrator3/1
  Integrator3/1 -> Saturation/1
  Subtract1/1 -> Integrator2/1
  Product3/1 -> Subtract1/1
  X Acceleration [m/s^2]/1 -> Add2/1
  Integrator4/1 -> To Workspace2/1, Yaw Rate/1, Product2/1, Product3/2  "Yaw_Rate [rad/s]"
  [V_x] -> Product3/1
  [V_y] -> Product2/2
  Saturation/1 -> To Workspace1/1, [V_x], X Velocity/1  "X Velocity [m/s]"

== system Rebuild/Main/Powertrain/Energy Calculation ==
  Motor Power [W] : Inport
  Add : Sum  Inputs=4
  Bus Selector : BusSelector  OutputSignals=Motor Power FL [W],Motor Power FR [W],Motor Power RL [W],Motor Power RR [W]
  Gain1 : Gain  Gain=1/3.6e6
  Integrator : Integrator
  Terminator : Terminator
  wires:
  Integrator/1 -> Gain1/1  "Energy [J]"
  Motor Power [W]/1 -> Bus Selector/1
  Bus Selector/1 -> Add/1  "<Motor Power FL [W]>"
  Bus Selector/2 -> Add/2  "<Motor Power FR [W]>"
  Bus Selector/3 -> Add/3  "<Motor Power RL [W]>"
  Bus Selector/4 -> Add/4  "<Motor Power RR [W]>"
  Add/1 -> Integrator/1  "Total Power [W]"
  Gain1/1 -> Terminator/1  "Energy Used [kWh]"

== system Rebuild/Main/Powertrain/Motors ==
  Add : Sum
  Bus Selector1 : BusSelector  OutputSignals=APPS [%],Brake Pressure [bar]
  Control Algorithms : Subsystem
  Field Weakening : Subsystem
  Power Limit : Subsystem
  Regen Braking : Subsystem
  Torque Command [Nm] : Subsystem
  Motor Torque [Nm] : Outport
  Motor Power [W] : Outport  Port=2
  wires:
  Field Weakening/1(Motor Torque after FW [Nm]) -> Control Algorithms/1(Motor Torque after FW [Nm])
  Control Algorithms/1(Motor Torque after TV [Nm]) -> Power Limit/1(Motor Torque after TV [Nm])
  Bus Selector1/2 -> Regen Braking/1(Brake Pressure [bar])  "<Brake Pressure [bar]>"
  Bus Selector1/1 -> Torque Command [Nm]/1(APPS)  "<APPS [%]>"
  [Driver_Inputs] -> Bus Selector1/1
  Torque Command [Nm]/1(Positive Torque Command [Nm]) -> Add/1
  Regen Braking/1(Negative Torque Command [Nm]) -> Add/2
  Add/1 -> Field Weakening/1(Requested_Motor_Torque)  "Torque Command {Nm]"
  Power Limit/2(Motor Torque [Nm]) -> Motor Torque [Nm]/1
  Power Limit/1(Motor Power [W]) -> Motor Power [W]/1

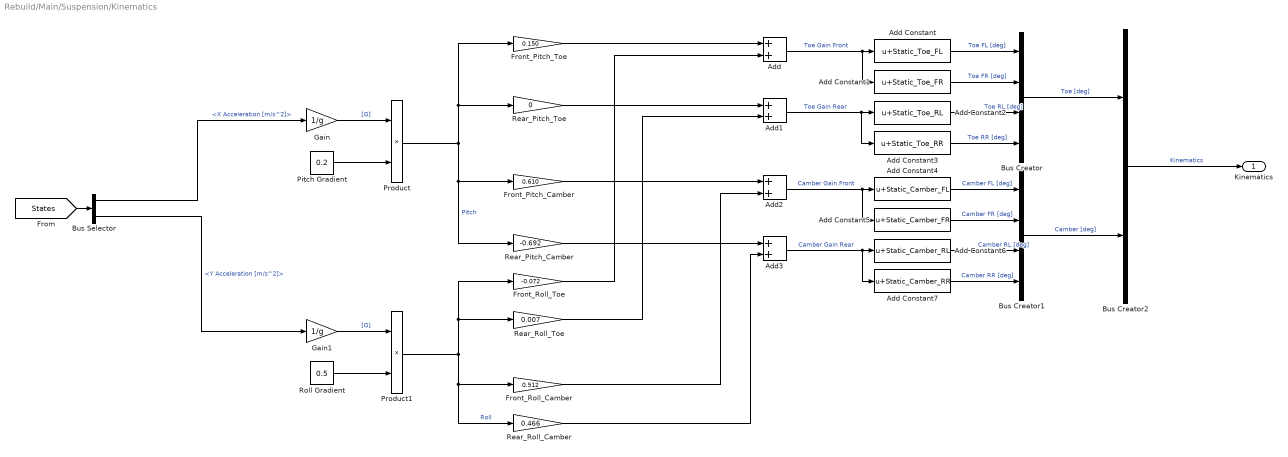
== system Rebuild/Main/Suspension/Kinematics ==
  Add{,1..3} (4 alike) : Sum
  Add Constant : Bias  Bias=Static_Toe_FL  SaturateOnIntegerOverflow=off
  Add Constant1 : Bias  Bias=Static_Toe_FR  SaturateOnIntegerOverflow=off
  Add Constant2 : Bias  Bias=Static_Toe_RL  SaturateOnIntegerOverflow=off
  Add Constant3 : Bias  Bias=Static_Toe_RR  SaturateOnIntegerOverflow=off
  Add Constant4 : Bias  Bias=Static_Camber_FL  SaturateOnIntegerOverflow=off
  Add Constant5 : Bias  Bias=Static_Camber_FR  SaturateOnIntegerOverflow=off
  Add Constant6 : Bias  Bias=Static_Camber_RL  SaturateOnIntegerOverflow=off
  Add Constant7 : Bias  Bias=Static_Camber_RR  SaturateOnIntegerOverflow=off
  Bus Creator : BusCreator  Inputs=4
  Bus Creator1 : BusCreator  Inputs=4
  Bus Creator2 : BusCreator  Inputs=2
  Bus Selector : BusSelector  OutputSignals=Acceleration [m/s].X Acceleration [m/s^2],Acceleration [m/s].Y Acceleration [m/s^2]
  Front_Pitch_Camber : Gain  Gain=0.610
  Front_Pitch_Toe : Gain  Gain=0.150
  Front_Roll_Camber : Gain  Gain=0.512
  Front_Roll_Toe : Gain  Gain=-0.072
  Gain : Gain  Gain=1/g
  Gain1 : Gain  Gain=1/g
  Pitch Gradient : Constant  Value=0.2
  Product : Product
  Product1 : Product
  Rear_Pitch_Camber : Gain  Gain=-0.692
  Rear_Pitch_Toe : Gain  Gain=0
  Rear_Roll_Camber : Gain  Gain=0.466
  Rear_Roll_Toe : Gain  Gain=0.007
  Roll Gradient : Constant  Value=0.5
  Kinematics : Outport
  wires:
  Rear_Pitch_Camber/1 -> Add3/1
  Front_Roll_Camber/1 -> Add2/2
  Rear_Pitch_Toe/1 -> Add1/1
  Front_Roll_Toe/1 -> Add/2
  Rear_Roll_Toe/1 -> Add1/2
  Gain/1 -> Product/1  "[G]"
  Product1/1 -> Rear_Roll_Toe/1, Front_Roll_Toe/1, Rear_Roll_Camber/1, Front_Roll_Camber/1  "Roll"
  Product/1 -> Rear_Pitch_Toe/1, Front_Pitch_Toe/1, Front_Pitch_Camber/1, Rear_Pitch_Camber/1  "Pitch"
  Front_Pitch_Toe/1 -> Add/1
  Rear_Roll_Camber/1 -> Add3/2
  Front_Pitch_Camber/1 -> Add2/1
  Gain1/1 -> Product1/1  "[G]"
  Pitch Gradient/1 -> Product/2
  Roll Gradient/1 -> Product1/2
  Bus Creator2/1 -> Kinematics/1  "Kinematics"
  Add1/1 -> Add Constant3/1, Add Constant2/1  "Toe Gain Rear"
  Add/1 -> Add Constant1/1, Add Constant/1  "Toe Gain Front"
  Add Constant/1 -> Bus Creator/1  "Toe FL [deg]"
  Add Constant1/1 -> Bus Creator/2  "Toe FR [deg]"
  Add Constant2/1 -> Bus Creator/3  "Toe RL [deg]"
  Add Constant3/1 -> Bus Creator/4  "Toe RR [deg]"
  Bus Creator/1 -> Bus Creator2/1  "Toe [deg]"
  Bus Creator1/1 -> Bus Creator2/2  "Camber [deg]"
  Add Constant7/1 -> Bus Creator1/4  "Camber RR [deg]"
  Add Constant6/1 -> Bus Creator1/3  "Camber RL [deg]"
  Add Constant5/1 -> Bus Creator1/2  "Camber FR [deg]"
  Add Constant4/1 -> Bus Creator1/1  "Camber FL [deg]"
  Add3/1 -> Add Constant7/1, Add Constant6/1  "Camber Gain Rear"
  Add2/1 -> Add Constant5/1, Add Constant4/1  "Camber Gain Front"
  [States] -> Bus Selector/1
  Bus Selector/1 -> Gain/1  "<X Acceleration [m/s^2]>"
  Bus Selector/2 -> Gain1/1  "<Y Acceleration [m/s^2]>"

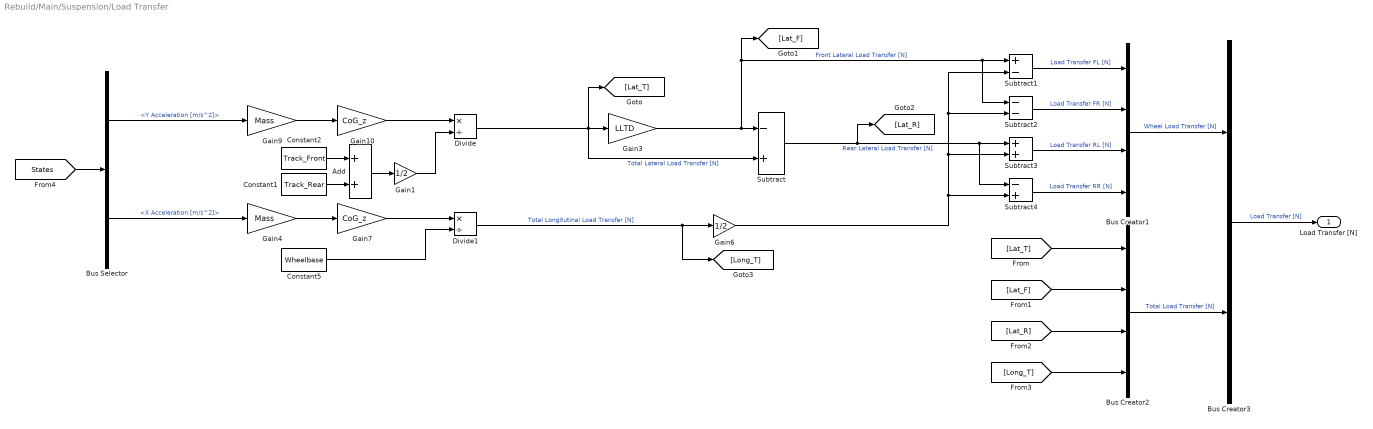
== system Rebuild/Main/Suspension/Load Transfer ==
  Add : Sum
  Bus Creator1 : BusCreator  Inputs=4
  Bus Creator2 : BusCreator  Inputs=4
  Bus Creator3 : BusCreator  Inputs=2
  Bus Selector : BusSelector  OutputSignals=Acceleration [m/s].Y Acceleration [m/s^2],Acceleration [m/s].X Acceleration [m/s^2]
  Constant1 : Constant  Value=Track_Rear
  Constant2 : Constant  Value=Track_Front
  Constant5 : Constant  Value=Wheelbase
  Divide : Product  Inputs=*/
  Divide1 : Product  Inputs=*/
  Gain1 : Gain  Gain=1/2
  Gain10 : Gain  Gain=CoG_z
  Gain3 : Gain  Gain=LLTD
  Gain4 : Gain  Gain=Mass
  Gain6 : Gain  Gain=1/2
  Gain7 : Gain  Gain=CoG_z
  Gain9 : Gain  Gain=Mass
  Subtract : Sum  Inputs=-+
  Subtract1 : Sum  Inputs=+-
  Subtract2 : Sum  Inputs=--
  Subtract3 : Sum
  Subtract4 : Sum  Inputs=-+
  Load Transfer [N] : Outport
  wires:
  [States] -> Bus Selector/1
  Gain1/1 -> Divide/2
  Constant2/1 -> Add/1
  Divide/1 -> [Lat_T], Subtract/2, Gain3/1  "Total Lateral Load Transfer [N]"
  Constant5/1 -> Divide1/2
  Divide1/1 -> [Long_T], Gain6/1  "Total Longitutinal Load Transfer [N]"
  Gain7/1 -> Divide1/1
  Bus Selector/1 -> Gain9/1  "<Y Acceleration [m/s^2]>"
  Gain9/1 -> Gain10/1
  Bus Selector/2 -> Gain4/1  "<X Acceleration [m/s^2]>"
  Gain4/1 -> Gain7/1
  Constant1/1 -> Add/2
  Add/1 -> Gain1/1
  Gain10/1 -> Divide/1
  Gain3/1 -> [Lat_F], Subtract1/1, Subtract2/1, Subtract/1  "Front Lateral Load Transfer [N]"
  Subtract/1 -> [Lat_R], Subtract4/1, Subtract3/1  "Rear Lateral Load Transfer [N]"
  Subtract1/1 -> Bus Creator1/1  "Load Transfer FL [N]"
  Gain6/1 -> Subtract4/2, Subtract1/2, Subtract2/2, Subtract3/2
  Subtract2/1 -> Bus Creator1/2  "Load Transfer FR [N]"
  Subtract3/1 -> Bus Creator1/3  "Load Transfer RL [N]"
  Subtract4/1 -> Bus Creator1/4  "Load Transfer RR [N]"
  [Lat_F] -> Bus Creator2/2
  [Long_T] -> Bus Creator2/4
  [Lat_T] -> Bus Creator2/1
  [Lat_R] -> Bus Creator2/3
  Bus Creator1/1 -> Bus Creator3/1  "Wheel Load Transfer [N]"
  Bus Creator2/1 -> Bus Creator3/2  "Total Load Transfer [N]"
  Bus Creator3/1 -> Load Transfer [N]/1  "Load Transfer [N]"

== system Rebuild/Main/Suspension/Steering ==
  Add : Sum
  Add1 : Sum
  Bus Creator : BusCreator  Inputs=4
  Bus Creator1 : BusCreator  Inputs=4
  Bus Selector : BusSelector  OutputSignals=Steering Position [deg]
  Bus Selector1 : BusSelector  OutputSignals=Kinematics.Toe [deg].Toe FL [deg],Kinematics.Toe [deg].Toe FR [deg],Kinematics.Toe [deg].Toe RL [deg],Kinematics.Toe [deg].Toe RR [deg]
  Degrees to Radians{,1..3} (4 alike) : simulink_extras/Transformations/Degrees to Radians
  FL : Lookup_n-D  NumberOfTableDimensions=1  BreakpointsForDimension1=Steering_Wheel_Angle  Table=Steering_Angle_FL  InternalRulePriority=Speed  RndMeth=Simplest
  FR : Lookup_n-D  NumberOfTableDimensions=1  BreakpointsForDimension1=Steering_Wheel_Angle  Table=Steering_Angle_FR*-1  InternalRulePriority=Speed  RndMeth=Simplest
  Terminator : Terminator
  Steering : Outport
  wires:
  Bus Creator/1 -> Steering/1  "Steering Angle [rad]"
  [Driver_Inputs] -> Bus Selector/1
  Bus Selector/1 -> FL/1, FR/1  "<Steering Position [deg]>"
  Degrees to Radians/1 -> Bus Creator/1  "Steering Angle FL [rad]"
  Degrees to Radians1/1 -> Bus Creator/2  "Steering Angle FR [rad]"
  Bus Creator1/1 -> Terminator/1  "Steering Angle [deg]"
  [Sus] -> Bus Selector1/1
  Bus Selector1/1 -> Add/2  "<Toe FL [deg]>"
  Bus Selector1/2 -> Add1/2  "<Toe FR [deg]>"
  Add/1 -> Degrees to Radians/1, Bus Creator1/1  "Steering Angle FL [deg]"
  Add1/1 -> Bus Creator1/2, Degrees to Radians1/1  "Steering Angle FR [deg]"
  Degrees to Radians2/1 -> Bus Creator/3  "Steering Angle RL [rad]"
  Degrees to Radians3/1 -> Bus Creator/4  "Steering Angle RR [rad]"
  Bus Selector1/3 -> Bus Creator1/3, Degrees to Radians2/1  "<Toe RL [deg]>"
  Bus Selector1/4 -> Bus Creator1/4, Degrees to Radians3/1  "<Toe RR [deg]>"
  FL/1 -> Add/1  "Steering Angle FL [deg]"
  FR/1 -> Add1/1  "Steering Angle FR [deg]"

== system Rebuild/Main/Wheels & Tires/Brakes ==
  Brake_Balance_Adjustment : Subsystem
  Braking_Torque_Front : Subsystem
  Braking_Torque_Rear : Subsystem
  Bus Creator2 : BusCreator  Inputs=4
  Bus Selector : BusSelector  OutputSignals=Brake Pressure [bar].Brake Pressure Front [bar],Brake Pressure [bar].Brake Pressure Rear [bar]
  Gain{,1..3} (4 alike) : Gain  Gain=0.5
  Brake Torque [Nm] : Outport
  wires:
  Bus Creator2/1 -> Brake Torque [Nm]/1  "Brake Torque [Nm]"
  Brake_Balance_Adjustment/1(Adj_Braking_Torque_F [Nm]) -> Gain1/1, Gain/1
  [Driver_Inputs] -> Bus Selector/1
  Brake_Balance_Adjustment/2(Adj_Braking_Torque_R [Nm]) -> Gain3/1, Gain2/1
  Braking_Torque_Front/1(Braking_torque [Nm]) -> Brake_Balance_Adjustment/1(Braking_Torque_F [Nm])
  Braking_Torque_Rear/1(Braking_Torque [Nm]) -> Brake_Balance_Adjustment/2(Braking_Torque_R [Nm])
  Bus Selector/1 -> Braking_Torque_Front/1(Brake_Pressure [bar])  "<Brake Pressure Front [bar]>"
  Bus Selector/2 -> Braking_Torque_Rear/1(Brake_Pressure [bar])  "<Brake Pressure Rear [bar]>"
  Gain/1 -> Bus Creator2/1  "Brake Torque FL [Nm]"
  Gain2/1 -> Bus Creator2/3  "Brake Torque RL [Nm]"
  Gain1/1 -> Bus Creator2/2  "Brake Torque FR [Nm]"
  Gain3/1 -> Bus Creator2/4  "Brake Torque RR [Nm]"
